simulink model "DriveSystemControl"  (R2023b)
settings: Solver=FixedStepAuto  StartTime=0.0  StopTime=Inf  FixedStep=0.001  RelTol=1e-3
PostLoadFcn:
  | if any(exist('dsrtsu_mdlpostloadfcn', 'file') ~= 0), dsrtsu_mdlpostloadfcn('Execute', bdroot); end
InitFcn:
  | , if any(exist('rtifpga_mdlclblib', 'file') ~= 0), rtifpga_mdlclblib('Init', bdroot); end,
  | , if any(exist('dsmpb_private', 'file') ~= 0), dsmpb_private('dsmpb_mdlclblib', 'Init', bdroot); end,
libraries: dsmpblib x2
(part 4 of 11)

== system DriveSystemControl/Bus Configuration (1) - In/Simulated ECUs/Virya Controller CAN File 08082024/TCU/TX/PDUs/TCU03/sigBPosUndervoltageCutback ==
  ISignal Value : Subsystem
  _sigBPosUndervoltageCutback_ : BusCreator  Inputs=1
  sigBPosUndervoltageCutback : Outport
  wires:
  _sigBPosUndervoltageCutback_/1 -> sigBPosUndervoltageCutback/1  "sigBPosUndervoltageCutback"
  ISignal Value/1(ISignal Value) -> _sigBPosUndervoltageCutback_/1  "ISignal Value"

== system DriveSystemControl/Bus Configuration (1) - In/Simulated ECUs/Virya Controller CAN File 08082024/TCU/TX/PDUs/TCU03/sigBadCalibration ==
  ISignal Value : Subsystem
  _sigBadCalibration_ : BusCreator  Inputs=1
  sigBadCalibration : Outport
  wires:
  _sigBadCalibration_/1 -> sigBadCalibration/1  "sigBadCalibration"
  ISignal Value/1(ISignal Value) -> _sigBadCalibration_/1  "ISignal Value"

== system DriveSystemControl/Bus Configuration (1) - In/Simulated ECUs/Virya Controller CAN File 08082024/TCU/TX/PDUs/TCU03/sigBrakeWiperHigh ==
  ISignal Value : Subsystem
  _sigBrakeWiperHigh_ : BusCreator  Inputs=1
  sigBrakeWiperHigh : Outport
  wires:
  _sigBrakeWiperHigh_/1 -> sigBrakeWiperHigh/1  "sigBrakeWiperHigh"
  ISignal Value/1(ISignal Value) -> _sigBrakeWiperHigh_/1  "ISignal Value"

== system DriveSystemControl/Bus Configuration (1) - In/Simulated ECUs/Virya Controller CAN File 08082024/TCU/TX/PDUs/TCU03/sigBrakeWiperLow ==
  ISignal Value : Subsystem
  _sigBrakeWiperLow_ : BusCreator  Inputs=1
  sigBrakeWiperLow : Outport
  wires:
  _sigBrakeWiperLow_/1 -> sigBrakeWiperLow/1  "sigBrakeWiperLow"
  ISignal Value/1(ISignal Value) -> _sigBrakeWiperLow_/1  "ISignal Value"

== system DriveSystemControl/Bus Configuration (1) - In/Simulated ECUs/Virya Controller CAN File 08082024/TCU/TX/PDUs/TCU03/sigCoil2DriverOpenShort ==
  ISignal Value : Subsystem
  _sigCoil2DriverOpenShort_ : BusCreator  Inputs=1
  sigCoil2DriverOpenShort : Outport
  wires:
  _sigCoil2DriverOpenShort_/1 -> sigCoil2DriverOpenShort/1  "sigCoil2DriverOpenShort"
  ISignal Value/1(ISignal Value) -> _sigCoil2DriverOpenShort_/1  "ISignal Value"

== system DriveSystemControl/Bus Configuration (1) - In/Simulated ECUs/Virya Controller CAN File 08082024/TCU/TX/PDUs/TCU03/sigCoil3DriverOpenShort ==
  ISignal Value : Subsystem
  _sigCoil3DriverOpenShort_ : BusCreator  Inputs=1
  sigCoil3DriverOpenShort : Outport
  wires:
  _sigCoil3DriverOpenShort_/1 -> sigCoil3DriverOpenShort/1  "sigCoil3DriverOpenShort"
  ISignal Value/1(ISignal Value) -> _sigCoil3DriverOpenShort_/1  "ISignal Value"

== system DriveSystemControl/Bus Configuration (1) - In/Simulated ECUs/Virya Controller CAN File 08082024/TCU/TX/PDUs/TCU03/sigCoil4DriverOpenShort ==
  ISignal Value : Subsystem
  _sigCoil4DriverOpenShort_ : BusCreator  Inputs=1
  sigCoil4DriverOpenShort : Outport
  wires:
  _sigCoil4DriverOpenShort_/1 -> sigCoil4DriverOpenShort/1  "sigCoil4DriverOpenShort"
  ISignal Value/1(ISignal Value) -> _sigCoil4DriverOpenShort_/1  "ISignal Value"

== system DriveSystemControl/Bus Configuration (1) - In/Simulated ECUs/Virya Controller CAN File 08082024/TCU/TX/PDUs/TCU03/sigControllerCommonFault ==
  ISignal Value : Subsystem
  _sigControllerCommonFault_ : BusCreator  Inputs=1
  sigControllerCommonFault : Outport
  wires:
  _sigControllerCommonFault_/1 -> sigControllerCommonFault/1  "sigControllerCommonFault"
  ISignal Value/1(ISignal Value) -> _sigControllerCommonFault_/1  "ISignal Value"

== system DriveSystemControl/Bus Configuration (1) - In/Simulated ECUs/Virya Controller CAN File 08082024/TCU/TX/PDUs/TCU03/sigControllerOverCurrent ==
  ISignal Value : Subsystem
  _sigControllerOverCurrent_ : BusCreator  Inputs=1
  sigControllerOverCurrent : Outport
  wires:
  _sigControllerOverCurrent_/1 -> sigControllerOverCurrent/1  "sigControllerOverCurrent"
  ISignal Value/1(ISignal Value) -> _sigControllerOverCurrent_/1  "ISignal Value"

== system DriveSystemControl/Bus Configuration (1) - In/Simulated ECUs/Virya Controller CAN File 08082024/TCU/TX/PDUs/TCU03/sigControllerOvertempCutback ==
  ISignal Value : Subsystem
  _sigControllerOvertempCutback_ : BusCreator  Inputs=1
  sigControllerOvertempCutback : Outport
  wires:
  _sigControllerOvertempCutback_/1 -> sigControllerOvertempCutback/1  "sigControllerOvertempCutback"
  ISignal Value/1(ISignal Value) -> _sigControllerOvertempCutback_/1  "ISignal Value"

== system DriveSystemControl/Bus Configuration (1) - In/Simulated ECUs/Virya Controller CAN File 08082024/TCU/TX/PDUs/TCU03/sigControllerSevereOvertemp ==
  ISignal Value : Subsystem
  _sigControllerSevereOvertemp_ : BusCreator  Inputs=1
  sigControllerSevereOvertemp : Outport
  wires:
  _sigControllerSevereOvertemp_/1 -> sigControllerSevereOvertemp/1  "sigControllerSevereOvertemp"
  ISignal Value/1(ISignal Value) -> _sigControllerSevereOvertemp_/1  "ISignal Value"

== system DriveSystemControl/Bus Configuration (1) - In/Simulated ECUs/Virya Controller CAN File 08082024/TCU/TX/PDUs/TCU03/sigControllerSevereUndertemp ==
  ISignal Value : Subsystem
  _sigControllerSevereUndertemp_ : BusCreator  Inputs=1
  sigControllerSevereUndertemp : Outport
  wires:
  _sigControllerSevereUndertemp_/1 -> sigControllerSevereUndertemp/1  "sigControllerSevereUndertemp"
  ISignal Value/1(ISignal Value) -> _sigControllerSevereUndertemp_/1  "ISignal Value"

== system DriveSystemControl/Bus Configuration (1) - In/Simulated ECUs/Virya Controller CAN File 08082024/TCU/TX/PDUs/TCU03/sigCurrentSensorFault ==
  ISignal Value : Subsystem
  _sigCurrentSensorFault_ : BusCreator  Inputs=1
  sigCurrentSensorFault : Outport
  wires:
  _sigCurrentSensorFault_/1 -> sigCurrentSensorFault/1  "sigCurrentSensorFault"
  ISignal Value/1(ISignal Value) -> _sigCurrentSensorFault_/1  "ISignal Value"

== system DriveSystemControl/Bus Configuration (1) - In/Simulated ECUs/Virya Controller CAN File 08082024/TCU/TX/PDUs/TCU03/sigEEPROMFailure ==
  ISignal Value : Subsystem
  _sigEEPROMFailure_ : BusCreator  Inputs=1
  sigEEPROMFailure : Outport
  wires:
  _sigEEPROMFailure_/1 -> sigEEPROMFailure/1  "sigEEPROMFailure"
  ISignal Value/1(ISignal Value) -> _sigEEPROMFailure_/1  "ISignal Value"

== system DriveSystemControl/Bus Configuration (1) - In/Simulated ECUs/Virya Controller CAN File 08082024/TCU/TX/PDUs/TCU03/sigHighPedalDisable ==
  ISignal Value : Subsystem
  _sigHighPedalDisable_ : BusCreator  Inputs=1
  sigHighPedalDisable : Outport
  wires:
  _sigHighPedalDisable_/1 -> sigHighPedalDisable/1  "sigHighPedalDisable"
  ISignal Value/1(ISignal Value) -> _sigHighPedalDisable_/1  "ISignal Value"

== system DriveSystemControl/Bus Configuration (1) - In/Simulated ECUs/Virya Controller CAN File 08082024/TCU/TX/PDUs/TCU03/sigInsulationResistanceLow ==
  ISignal Value : Subsystem
  _sigInsulationResistanceLow_ : BusCreator  Inputs=1
  sigInsulationResistanceLow : Outport
  wires:
  _sigInsulationResistanceLow_/1 -> sigInsulationResistanceLow/1  "sigInsulationResistanceLow"
  ISignal Value/1(ISignal Value) -> _sigInsulationResistanceLow_/1  "ISignal Value"

== system DriveSystemControl/Bus Configuration (1) - In/Simulated ECUs/Virya Controller CAN File 08082024/TCU/TX/PDUs/TCU03/sigMainContactorWelded ==
  ISignal Value : Subsystem
  _sigMainContactorWelded_ : BusCreator  Inputs=1
  sigMainContactorWelded : Outport
  wires:
  _sigMainContactorWelded_/1 -> sigMainContactorWelded/1  "sigMainContactorWelded"
  ISignal Value/1(ISignal Value) -> _sigMainContactorWelded_/1  "ISignal Value"

== system DriveSystemControl/Bus Configuration (1) - In/Simulated ECUs/Virya Controller CAN File 08082024/TCU/TX/PDUs/TCU03/sigMainContactordidnotClose ==
  ISignal Value : Subsystem
  _sigMainContactordidnotClose_ : BusCreator  Inputs=1
  sigMainContactordidnotClose : Outport
  wires:
  _sigMainContactordidnotClose_/1 -> sigMainContactordidnotClose/1  "sigMainContactordidnotClose"
  ISignal Value/1(ISignal Value) -> _sigMainContactordidnotClose_/1  "ISignal Value"

== system DriveSystemControl/Bus Configuration (1) - In/Simulated ECUs/Virya Controller CAN File 08082024/TCU/TX/PDUs/TCU03/sigMainOpenShort ==
  ISignal Value : Subsystem
  _sigMainOpenShort_ : BusCreator  Inputs=1
  sigMainOpenShort : Outport
  wires:
  _sigMainOpenShort_/1 -> sigMainOpenShort/1  "sigMainOpenShort"
  ISignal Value/1(ISignal Value) -> _sigMainOpenShort_/1  "ISignal Value"

== system DriveSystemControl/Bus Configuration (1) - In/Simulated ECUs/Virya Controller CAN File 08082024/TCU/TX/PDUs/TCU03/sigMotorCharacterization ==
  ISignal Value : Subsystem
  _sigMotorCharacterization_ : BusCreator  Inputs=1
  sigMotorCharacterization : Outport
  wires:
  _sigMotorCharacterization_/1 -> sigMotorCharacterization/1  "sigMotorCharacterization"
  ISignal Value/1(ISignal Value) -> _sigMotorCharacterization_/1  "ISignal Value"

== system DriveSystemControl/Bus Configuration (1) - In/Simulated ECUs/Virya Controller CAN File 08082024/TCU/TX/PDUs/TCU03/sigMotorPhaseOpen ==
  ISignal Value : Subsystem
  _sigMotorPhaseOpen_ : BusCreator  Inputs=1
  sigMotorPhaseOpen : Outport
  wires:
  _sigMotorPhaseOpen_/1 -> sigMotorPhaseOpen/1  "sigMotorPhaseOpen"
  ISignal Value/1(ISignal Value) -> _sigMotorPhaseOpen_/1  "ISignal Value"

== system DriveSystemControl/Bus Configuration (1) - In/Simulated ECUs/Virya Controller CAN File 08082024/TCU/TX/PDUs/TCU03/sigMotorTempHotCutback ==
  ISignal Value : Subsystem
  _sigMotorTempHotCutback_ : BusCreator  Inputs=1
  sigMotorTempHotCutback : Outport
  wires:
  _sigMotorTempHotCutback_/1 -> sigMotorTempHotCutback/1  "sigMotorTempHotCutback"
  ISignal Value/1(ISignal Value) -> _sigMotorTempHotCutback_/1  "ISignal Value"

== system DriveSystemControl/Bus Configuration (1) - In/Simulated ECUs/Virya Controller CAN File 08082024/TCU/TX/PDUs/TCU03/sigMotorTempSensorFault ==
  ISignal Value : Subsystem
  _sigMotorTempSensorFault_ : BusCreator  Inputs=1
  sigMotorTempSensorFault : Outport
  wires:
  _sigMotorTempSensorFault_/1 -> sigMotorTempSensorFault/1  "sigMotorTempSensorFault"
  ISignal Value/1(ISignal Value) -> _sigMotorTempSensorFault_/1  "ISignal Value"

== system DriveSystemControl/Bus Configuration (1) - In/Simulated ECUs/Virya Controller CAN File 08082024/TCU/TX/PDUs/TCU03/sigOEM_BatterySTOPSignal ==
  ISignal Value : Subsystem
  _sigOEM_BatterySTOPSignal_ : BusCreator  Inputs=1
  sigOEM_BatterySTOPSignal : Outport
  wires:
  _sigOEM_BatterySTOPSignal_/1 -> sigOEM_BatterySTOPSignal/1  "sigOEM_BatterySTOPSignal"
  ISignal Value/1(ISignal Value) -> _sigOEM_BatterySTOPSignal_/1  "ISignal Value"

== system DriveSystemControl/Bus Configuration (1) - In/Simulated ECUs/Virya Controller CAN File 08082024/TCU/TX/PDUs/TCU03/sigOEM_NoBatteryCAN ==
  ISignal Value : Subsystem
  _sigOEM_NoBatteryCAN_ : BusCreator  Inputs=1
  sigOEM_NoBatteryCAN : Outport
  wires:
  _sigOEM_NoBatteryCAN_/1 -> sigOEM_NoBatteryCAN/1  "sigOEM_NoBatteryCAN"
  ISignal Value/1(ISignal Value) -> _sigOEM_NoBatteryCAN_/1  "ISignal Value"

== system DriveSystemControl/Bus Configuration (1) - In/Simulated ECUs/Virya Controller CAN File 08082024/TCU/TX/PDUs/TCU03/sigOSGeneral ==
  ISignal Value : Subsystem
  _sigOSGeneral_ : BusCreator  Inputs=1
  sigOSGeneral : Outport
  wires:
  _sigOSGeneral_/1 -> sigOSGeneral/1  "sigOSGeneral"
  ISignal Value/1(ISignal Value) -> _sigOSGeneral_/1  "ISignal Value"

== system DriveSystemControl/Bus Configuration (1) - In/Simulated ECUs/Virya Controller CAN File 08082024/TCU/TX/PDUs/TCU03/sigPMACCommissioningNeeded ==
  ISignal Value : Subsystem
  _sigPMACCommissioningNeeded_ : BusCreator  Inputs=1
  sigPMACCommissioningNeeded : Outport
  wires:
  _sigPMACCommissioningNeeded_/1 -> sigPMACCommissioningNeeded/1  "sigPMACCommissioningNeeded"
  ISignal Value/1(ISignal Value) -> _sigPMACCommissioningNeeded_/1  "ISignal Value"

== system DriveSystemControl/Bus Configuration (1) - In/Simulated ECUs/Virya Controller CAN File 08082024/TCU/TX/PDUs/TCU03/sigParameterChangeFault ==
  ISignal Value : Subsystem
  _sigParameterChangeFault_ : BusCreator  Inputs=1
  sigParameterChangeFault : Outport
  wires:
  _sigParameterChangeFault_/1 -> sigParameterChangeFault/1  "sigParameterChangeFault"
  ISignal Value/1(ISignal Value) -> _sigParameterChangeFault_/1  "ISignal Value"

== system DriveSystemControl/Bus Configuration (1) - In/Simulated ECUs/Virya Controller CAN File 08082024/TCU/TX/PDUs/TCU03/sigPhasePWMMismatch ==
  ISignal Value : Subsystem
  _sigPhasePWMMismatch_ : BusCreator  Inputs=1
  sigPhasePWMMismatch : Outport
  wires:
  _sigPhasePWMMismatch_/1 -> sigPhasePWMMismatch/1  "sigPhasePWMMismatch"
  ISignal Value/1(ISignal Value) -> _sigPhasePWMMismatch_/1  "ISignal Value"

== system DriveSystemControl/Bus Configuration (1) - In/Simulated ECUs/Virya Controller CAN File 08082024/TCU/TX/PDUs/TCU03/sigPrechargeFailed ==
  ISignal Value : Subsystem
  _sigPrechargeFailed_ : BusCreator  Inputs=1
  sigPrechargeFailed : Outport
  wires:
  _sigPrechargeFailed_/1 -> sigPrechargeFailed/1  "sigPrechargeFailed"
  ISignal Value/1(ISignal Value) -> _sigPrechargeFailed_/1  "ISignal Value"

== system DriveSystemControl/Bus Configuration (1) - In/Simulated ECUs/Virya Controller CAN File 08082024/TCU/TX/PDUs/TCU03/sigSevereBPosOvervoltage ==
  ISignal Value : Subsystem
  _sigSevereBPosOvervoltage_ : BusCreator  Inputs=1
  sigSevereBPosOvervoltage : Outport
  wires:
  _sigSevereBPosOvervoltage_/1 -> sigSevereBPosOvervoltage/1  "sigSevereBPosOvervoltage"
  ISignal Value/1(ISignal Value) -> _sigSevereBPosOvervoltage_/1  "ISignal Value"

== system DriveSystemControl/Bus Configuration (1) - In/Simulated ECUs/Virya Controller CAN File 08082024/TCU/TX/PDUs/TCU03/sigSevereBPosUndervoltage ==
  ISignal Value : Subsystem
  _sigSevereBPosUndervoltage_ : BusCreator  Inputs=1
  sigSevereBPosUndervoltage : Outport
  wires:
  _sigSevereBPosUndervoltage_/1 -> sigSevereBPosUndervoltage/1  "sigSevereBPosUndervoltage"
  ISignal Value/1(ISignal Value) -> _sigSevereBPosUndervoltage_/1  "ISignal Value"

== system DriveSystemControl/Bus Configuration (1) - In/Simulated ECUs/Virya Controller CAN File 08082024/TCU/TX/PDUs/TCU03/sigSevereKSIOvervoltage ==
  ISignal Value : Subsystem
  _sigSevereKSIOvervoltage_ : BusCreator  Inputs=1
  sigSevereKSIOvervoltage : Outport
  wires:
  _sigSevereKSIOvervoltage_/1 -> sigSevereKSIOvervoltage/1  "sigSevereKSIOvervoltage"
  ISignal Value/1(ISignal Value) -> _sigSevereKSIOvervoltage_/1  "ISignal Value"

== system DriveSystemControl/Bus Configuration (1) - In/Simulated ECUs/Virya Controller CAN File 08082024/TCU/TX/PDUs/TCU03/sigSevereKSIUndervoltage ==
  ISignal Value : Subsystem
  _sigSevereKSIUndervoltage_ : BusCreator  Inputs=1
  sigSevereKSIUndervoltage : Outport
  wires:
  _sigSevereKSIUndervoltage_/1 -> sigSevereKSIUndervoltage/1  "sigSevereKSIUndervoltage"
  ISignal Value/1(ISignal Value) -> _sigSevereKSIUndervoltage_/1  "ISignal Value"

== system DriveSystemControl/Bus Configuration (1) - In/Simulated ECUs/Virya Controller CAN File 08082024/TCU/TX/PDUs/TCU03/sigSinCosMisalignment ==
  ISignal Value : Subsystem
  _sigSinCosMisalignment_ : BusCreator  Inputs=1
  sigSinCosMisalignment : Outport
  wires:
  _sigSinCosMisalignment_/1 -> sigSinCosMisalignment/1  "sigSinCosMisalignment"
  ISignal Value/1(ISignal Value) -> _sigSinCosMisalignment_/1  "ISignal Value"

== system DriveSystemControl/Bus Configuration (1) - In/Simulated ECUs/Virya Controller CAN File 08082024/TCU/TX/PDUs/TCU03/sigSinCosSensorFault ==
  ISignal Value : Subsystem
  _sigSinCosSensorFault_ : BusCreator  Inputs=1
  sigSinCosSensorFault : Outport
  wires:
  _sigSinCosSensorFault_/1 -> sigSinCosSensorFault/1  "sigSinCosSensorFault"
  ISignal Value/1(ISignal Value) -> _sigSinCosSensorFault_/1  "ISignal Value"

== system DriveSystemControl/Bus Configuration (1) - In/Simulated ECUs/Virya Controller CAN File 08082024/TCU/TX/PDUs/TCU03/sigStallDetected ==
  ISignal Value : Subsystem
  _sigStallDetected_ : BusCreator  Inputs=1
  sigStallDetected : Outport
  wires:
  _sigStallDetected_/1 -> sigStallDetected/1  "sigStallDetected"
  ISignal Value/1(ISignal Value) -> _sigStallDetected_/1  "ISignal Value"

== system DriveSystemControl/Bus Configuration (1) - In/Simulated ECUs/Virya Controller CAN File 08082024/TCU/TX/PDUs/TCU03/sigSupervisorFault ==
  ISignal Value : Subsystem
  _sigSupervisorFault_ : BusCreator  Inputs=1
  sigSupervisorFault : Outport
  wires:
  _sigSupervisorFault_/1 -> sigSupervisorFault/1  "sigSupervisorFault"
  ISignal Value/1(ISignal Value) -> _sigSupervisorFault_/1  "ISignal Value"

== system DriveSystemControl/Bus Configuration (1) - In/Simulated ECUs/Virya Controller CAN File 08082024/TCU/TX/PDUs/TCU03/sigThrottlewiperHigh ==
  ISignal Value : Subsystem
  _sigThrottlewiperHigh_ : BusCreator  Inputs=1
  sigThrottlewiperHigh : Outport
  wires:
  _sigThrottlewiperHigh_/1 -> sigThrottlewiperHigh/1  "sigThrottlewiperHigh"
  ISignal Value/1(ISignal Value) -> _sigThrottlewiperHigh_/1  "ISignal Value"

== system DriveSystemControl/Bus Configuration (1) - In/Simulated ECUs/Virya Controller CAN File 08082024/TCU/TX/PDUs/TCU03/sigThrottlewiperLow ==
  ISignal Value : Subsystem
  _sigThrottlewiperLow_ : BusCreator  Inputs=1
  sigThrottlewiperLow : Outport
  wires:
  _sigThrottlewiperLow_/1 -> sigThrottlewiperLow/1  "sigThrottlewiperLow"
  ISignal Value/1(ISignal Value) -> _sigThrottlewiperLow_/1  "ISignal Value"

== system DriveSystemControl/Bus Configuration (1) - In/Simulated ECUs/Virya Controller CAN File 08082024/TCU/TX/PDUs/TCU03/sigVCLRunTimeError ==
  ISignal Value : Subsystem
  _sigVCLRunTimeError_ : BusCreator  Inputs=1
  sigVCLRunTimeError : Outport
  wires:
  _sigVCLRunTimeError_/1 -> sigVCLRunTimeError/1  "sigVCLRunTimeError"
  ISignal Value/1(ISignal Value) -> _sigVCLRunTimeError_/1  "ISignal Value"

== system DriveSystemControl/Bus Configuration (1) - In/Simulated ECUs/Virya Controller CAN File 08082024/TCU/TX/PDUs/TCU04/sigMCU5_DriveMode ==
  ISignal Value : Subsystem
  _sigMCU5_DriveMode_ : BusCreator  Inputs=1
  sigMCU5_DriveMode : Outport
  wires:
  _sigMCU5_DriveMode_/1 -> sigMCU5_DriveMode/1  "sigMCU5_DriveMode"
  ISignal Value/1(ISignal Value) -> _sigMCU5_DriveMode_/1  "ISignal Value"

== system DriveSystemControl/Bus Configuration (1) - In/Simulated ECUs/Virya Controller CAN File 08082024/TCU/TX/PDUs/TCU04/sigMCU5_Efficiency ==
  ISignal Value : Subsystem
  _sigMCU5_Efficiency_ : BusCreator  Inputs=1
  sigMCU5_Efficiency : Outport
  wires:
  _sigMCU5_Efficiency_/1 -> sigMCU5_Efficiency/1  "sigMCU5_Efficiency"
  ISignal Value/1(ISignal Value) -> _sigMCU5_Efficiency_/1  "ISignal Value"

== system DriveSystemControl/Bus Configuration (1) - In/Simulated ECUs/Virya Controller CAN File 08082024/TCU/TX/PDUs/TCU04/sigMCU5_Hillhold ==
  ISignal Value : Subsystem
  _sigMCU5_Hillhold_ : BusCreator  Inputs=1
  sigMCU5_Hillhold : Outport
  wires:
  _sigMCU5_Hillhold_/1 -> sigMCU5_Hillhold/1  "sigMCU5_Hillhold"
  ISignal Value/1(ISignal Value) -> _sigMCU5_Hillhold_/1  "ISignal Value"

== system DriveSystemControl/Bus Configuration (1) - In/Simulated ECUs/Virya Controller CAN File 08082024/TCU/TX/PDUs/TCU04/sigMCU5_RegenFlag ==
  ISignal Value : Subsystem
  _sigMCU5_RegenFlag_ : BusCreator  Inputs=1
  sigMCU5_RegenFlag : Outport
  wires:
  _sigMCU5_RegenFlag_/1 -> sigMCU5_RegenFlag/1  "sigMCU5_RegenFlag"
  ISignal Value/1(ISignal Value) -> _sigMCU5_RegenFlag_/1  "ISignal Value"

== system DriveSystemControl/Bus Configuration (1) - In/Simulated ECUs/Virya Controller CAN File 08082024/TCU/TX/PDUs/TCU04/sigMCU5_Speed ==
  ISignal Value : Subsystem
  _sigMCU5_Speed_ : BusCreator  Inputs=1
  sigMCU5_Speed : Outport
  wires:
  _sigMCU5_Speed_/1 -> sigMCU5_Speed/1  "sigMCU5_Speed"
  ISignal Value/1(ISignal Value) -> _sigMCU5_Speed_/1  "ISignal Value"

== system DriveSystemControl/Bus Configuration (1) - In/Simulated ECUs/Virya Controller CAN File 08082024/TCU/TX/PDUs/TCU05/sigMCU6_Odometer ==
  ISignal Value : Subsystem
  _sigMCU6_Odometer_ : BusCreator  Inputs=1
  sigMCU6_Odometer : Outport
  wires:
  _sigMCU6_Odometer_/1 -> sigMCU6_Odometer/1  "sigMCU6_Odometer"
  ISignal Value/1(ISignal Value) -> _sigMCU6_Odometer_/1  "ISignal Value"

== system DriveSystemControl/Bus Configuration (1) - Out/Manipulation/Virya Controller CAN File 08082024/WIP/CANChannel/PDUs/BMS01/sigBatteryMalfunctionLight ==
  sigBatteryMalfunctionLight : Inport
  Feature Switch : Subsystem
  _sigBatteryMalfunctionLight_ : BusSelector  OutputSignals=Feature Switch
  wires:
  sigBatteryMalfunctionLight/1 -> _sigBatteryMalfunctionLight_/1  "sigBatteryMalfunctionLight"
  _sigBatteryMalfunctionLight_/1 -> Feature Switch/1(Feature Switch)  "<Feature Switch>"

== system DriveSystemControl/Bus Configuration (1) - Out/Manipulation/Virya Controller CAN File 08082024/WIP/CANChannel/PDUs/BMS01/sigKeyOnIndicator ==
  sigKeyOnIndicator : Inport
  Feature Switch : Subsystem
  _sigKeyOnIndicator_ : BusSelector  OutputSignals=Feature Switch
  wires:
  sigKeyOnIndicator/1 -> _sigKeyOnIndicator_/1  "sigKeyOnIndicator"
  _sigKeyOnIndicator_/1 -> Feature Switch/1(Feature Switch)  "<Feature Switch>"

== system DriveSystemControl/Bus Configuration (1) - Out/Manipulation/Virya Controller CAN File 08082024/WIP/CANChannel/PDUs/BMS01/sigStateOfCharge ==
  sigStateOfCharge : Inport
  Feature Switch : Subsystem
  _sigStateOfCharge_ : BusSelector  OutputSignals=Feature Switch
  wires:
  sigStateOfCharge/1 -> _sigStateOfCharge_/1  "sigStateOfCharge"
  _sigStateOfCharge_/1 -> Feature Switch/1(Feature Switch)  "<Feature Switch>"

== system DriveSystemControl/Bus Configuration (1) - Out/Manipulation/Virya Controller CAN File 08082024/WIP/CANChannel/PDUs/BMS02/sigBatteryCurrent ==
  sigBatteryCurrent : Inport
  Feature Switch : Subsystem
  _sigBatteryCurrent_ : BusSelector  OutputSignals=Feature Switch
  wires:
  sigBatteryCurrent/1 -> _sigBatteryCurrent_/1  "sigBatteryCurrent"
  _sigBatteryCurrent_/1 -> Feature Switch/1(Feature Switch)  "<Feature Switch>"

== system DriveSystemControl/Bus Configuration (1) - Out/Manipulation/Virya Controller CAN File 08082024/WIP/CANChannel/PDUs/BMS02/sigDriveCurrentLimit ==
  sigDriveCurrentLimit : Inport
  Feature Switch : Subsystem
  _sigDriveCurrentLimit_ : BusSelector  OutputSignals=Feature Switch
  wires:
  sigDriveCurrentLimit/1 -> _sigDriveCurrentLimit_/1  "sigDriveCurrentLimit"
  _sigDriveCurrentLimit_/1 -> Feature Switch/1(Feature Switch)  "<Feature Switch>"

== system DriveSystemControl/Bus Configuration (1) - Out/Manipulation/Virya Controller CAN File 08082024/WIP/CANChannel/PDUs/BMS02/sigRegenCurrentLimit ==
  sigRegenCurrentLimit : Inport
  Feature Switch : Subsystem
  _sigRegenCurrentLimit_ : BusSelector  OutputSignals=Feature Switch
  wires:
  sigRegenCurrentLimit/1 -> _sigRegenCurrentLimit_/1  "sigRegenCurrentLimit"
  _sigRegenCurrentLimit_/1 -> Feature Switch/1(Feature Switch)  "<Feature Switch>"

== system DriveSystemControl/Bus Configuration (1) - Out/Manipulation/Virya Controller CAN File 08082024/WIP/CANChannel/PDUs/BMS02/sigVehicleModeRequest ==
  sigVehicleModeRequest : Inport
  Feature Switch : Subsystem
  _sigVehicleModeRequest_ : BusSelector  OutputSignals=Feature Switch
  wires:
  sigVehicleModeRequest/1 -> _sigVehicleModeRequest_/1  "sigVehicleModeRequest"
  _sigVehicleModeRequest_/1 -> Feature Switch/1(Feature Switch)  "<Feature Switch>"

== system DriveSystemControl/Bus Configuration (1) - Out/Manipulation/Virya Controller CAN File 08082024/WIP/CANChannel/PDUs/MainController/CCU_heartBeat ==
  CCU_heartBeat : Inport
  Feature Switch : Subsystem
  _CCU_heartBeat_ : BusSelector  OutputSignals=Feature Switch
  wires:
  CCU_heartBeat/1 -> _CCU_heartBeat_/1  "CCU_heartBeat"
  _CCU_heartBeat_/1 -> Feature Switch/1(Feature Switch)  "<Feature Switch>"

== system DriveSystemControl/Bus Configuration (1) - Out/Manipulation/Virya Controller CAN File 08082024/WIP/CANChannel/PDUs/MainController/notUsed ==
  notUsed : Inport
  Feature Switch : Subsystem
  _notUsed_ : BusSelector  OutputSignals=Feature Switch
  wires:
  notUsed/1 -> _notUsed_/1  "notUsed"
  _notUsed_/1 -> Feature Switch/1(Feature Switch)  "<Feature Switch>"

== system DriveSystemControl/Bus Configuration (1) - Out/Manipulation/Virya Controller CAN File 08082024/WIP/CANChannel/PDUs/MainController/setAutoParkBreak ==
  setAutoParkBreak : Inport
  Feature Switch : Subsystem
  _setAutoParkBreak_ : BusSelector  OutputSignals=Feature Switch
  wires:
  setAutoParkBreak/1 -> _setAutoParkBreak_/1  "setAutoParkBreak"
  _setAutoParkBreak_/1 -> Feature Switch/1(Feature Switch)  "<Feature Switch>"

== system DriveSystemControl/Bus Configuration (1) - Out/Manipulation/Virya Controller CAN File 08082024/WIP/CANChannel/PDUs/MainController/setBreake ==
  setBreake : Inport
  Feature Switch : Subsystem
  _setBreake_ : BusSelector  OutputSignals=Feature Switch
  wires:
  setBreake/1 -> _setBreake_/1  "setBreake"
  _setBreake_/1 -> Feature Switch/1(Feature Switch)  "<Feature Switch>"

== system DriveSystemControl/Bus Configuration (1) - Out/Manipulation/Virya Controller CAN File 08082024/WIP/CANChannel/PDUs/MainController/setDirection ==
  setDirection : Inport
  Feature Switch : Subsystem
  _setDirection_ : BusSelector  OutputSignals=Feature Switch
  wires:
  setDirection/1 -> _setDirection_/1  "setDirection"
  _setDirection_/1 -> Feature Switch/1(Feature Switch)  "<Feature Switch>"

== system DriveSystemControl/Bus Configuration (1) - Out/Manipulation/Virya Controller CAN File 08082024/WIP/CANChannel/PDUs/MainController/setDriveMode ==
  setDriveMode : Inport
  Feature Switch : Subsystem
  _setDriveMode_ : BusSelector  OutputSignals=Feature Switch
  wires:
  setDriveMode/1 -> _setDriveMode_/1  "setDriveMode"
  _setDriveMode_/1 -> Feature Switch/1(Feature Switch)  "<Feature Switch>"

== system DriveSystemControl/Bus Configuration (1) - Out/Manipulation/Virya Controller CAN File 08082024/WIP/CANChannel/PDUs/MainController/setVelocity ==
  setVelocity : Inport
  Feature Switch : Subsystem
  _setVelocity_ : BusSelector  OutputSignals=Feature Switch
  wires:
  setVelocity/1 -> _setVelocity_/1  "setVelocity"
  _setVelocity_/1 -> Feature Switch/1(Feature Switch)  "<Feature Switch>"

== system DriveSystemControl/Bus Configuration (1) - Out/Manipulation/Virya Controller CAN File 08082024/WIP/CANChannel/PDUs/MainController/steeringPower ==
  steeringPower : Inport
  Feature Switch : Subsystem
  _steeringPower_ : BusSelector  OutputSignals=Feature Switch
  wires:
  steeringPower/1 -> _steeringPower_/1  "steeringPower"
  _steeringPower_/1 -> Feature Switch/1(Feature Switch)  "<Feature Switch>"

== system DriveSystemControl/Bus Configuration (1) - Out/Manipulation/Virya Controller CAN File 08082024/WIP/CANChannel/PDUs/TCU01/sigBrake ==
  sigBrake : Inport
  Feature Switch : Subsystem
  _sigBrake_ : BusSelector  OutputSignals=Feature Switch
  wires:
  sigBrake/1 -> _sigBrake_/1  "sigBrake"
  _sigBrake_/1 -> Feature Switch/1(Feature Switch)  "<Feature Switch>"

== system DriveSystemControl/Bus Configuration (1) - Out/Manipulation/Virya Controller CAN File 08082024/WIP/CANChannel/PDUs/TCU01/sigControllerTemperature ==
  sigControllerTemperature : Inport
  Feature Switch : Subsystem
  _sigControllerTemperature_ : BusSelector  OutputSignals=Feature Switch
  wires:
  sigControllerTemperature/1 -> _sigControllerTemperature_/1  "sigControllerTemperature"
  _sigControllerTemperature_/1 -> Feature Switch/1(Feature Switch)  "<Feature Switch>"

== system DriveSystemControl/Bus Configuration (1) - Out/Manipulation/Virya Controller CAN File 08082024/WIP/CANChannel/PDUs/TCU01/sigDriveMode ==
  sigDriveMode : Inport
  Feature Switch : Subsystem
  _sigDriveMode_ : BusSelector  OutputSignals=Feature Switch
  wires:
  sigDriveMode/1 -> _sigDriveMode_/1  "sigDriveMode"
  _sigDriveMode_/1 -> Feature Switch/1(Feature Switch)  "<Feature Switch>"

== system DriveSystemControl/Bus Configuration (1) - Out/Manipulation/Virya Controller CAN File 08082024/WIP/CANChannel/PDUs/TCU01/sigMotorTemperature ==
  sigMotorTemperature : Inport
  Feature Switch : Subsystem
  _sigMotorTemperature_ : BusSelector  OutputSignals=Feature Switch
  wires:
  sigMotorTemperature/1 -> _sigMotorTemperature_/1  "sigMotorTemperature"
  _sigMotorTemperature_/1 -> Feature Switch/1(Feature Switch)  "<Feature Switch>"

== system DriveSystemControl/Bus Configuration (1) - Out/Manipulation/Virya Controller CAN File 08082024/WIP/CANChannel/PDUs/TCU01/sigRMSCurrent ==
  sigRMSCurrent : Inport
  Feature Switch : Subsystem
  _sigRMSCurrent_ : BusSelector  OutputSignals=Feature Switch
  wires:
  sigRMSCurrent/1 -> _sigRMSCurrent_/1  "sigRMSCurrent"
  _sigRMSCurrent_/1 -> Feature Switch/1(Feature Switch)  "<Feature Switch>"

== system DriveSystemControl/Bus Configuration (1) - Out/Manipulation/Virya Controller CAN File 08082024/WIP/CANChannel/PDUs/TCU01/sigSpeed ==
  sigSpeed : Inport
  Feature Switch : Subsystem
  _sigSpeed_ : BusSelector  OutputSignals=Feature Switch
  wires:
  sigSpeed/1 -> _sigSpeed_/1  "sigSpeed"
  _sigSpeed_/1 -> Feature Switch/1(Feature Switch)  "<Feature Switch>"

== system DriveSystemControl/Bus Configuration (1) - Out/Manipulation/Virya Controller CAN File 08082024/WIP/CANChannel/PDUs/TCU01/sigThrottle ==
  sigThrottle : Inport
  Feature Switch : Subsystem
  _sigThrottle_ : BusSelector  OutputSignals=Feature Switch
  wires:
  sigThrottle/1 -> _sigThrottle_/1  "sigThrottle"
  _sigThrottle_/1 -> Feature Switch/1(Feature Switch)  "<Feature Switch>"

== system DriveSystemControl/Bus Configuration (1) - Out/Manipulation/Virya Controller CAN File 08082024/WIP/CANChannel/PDUs/TCU02/sigCapacitorVoltage ==
  sigCapacitorVoltage : Inport
  Feature Switch : Subsystem
  _sigCapacitorVoltage_ : BusSelector  OutputSignals=Feature Switch
  wires:
  sigCapacitorVoltage/1 -> _sigCapacitorVoltage_/1  "sigCapacitorVoltage"
  _sigCapacitorVoltage_/1 -> Feature Switch/1(Feature Switch)  "<Feature Switch>"

== system DriveSystemControl/Bus Configuration (1) - Out/Manipulation/Virya Controller CAN File 08082024/WIP/CANChannel/PDUs/TCU02/sigMotorRPM ==
  sigMotorRPM : Inport
  Feature Switch : Subsystem
  _sigMotorRPM_ : BusSelector  OutputSignals=Feature Switch
  wires:
  sigMotorRPM/1 -> _sigMotorRPM_/1  "sigMotorRPM"
  _sigMotorRPM_/1 -> Feature Switch/1(Feature Switch)  "<Feature Switch>"

== system DriveSystemControl/Bus Configuration (1) - Out/Manipulation/Virya Controller CAN File 08082024/WIP/CANChannel/PDUs/TCU02/sigOdometer ==
  sigOdometer : Inport
  Feature Switch : Subsystem
  _sigOdometer_ : BusSelector  OutputSignals=Feature Switch
  wires:
  sigOdometer/1 -> _sigOdometer_/1  "sigOdometer"
  _sigOdometer_/1 -> Feature Switch/1(Feature Switch)  "<Feature Switch>"

== system DriveSystemControl/Bus Configuration (1) - Out/Manipulation/Virya Controller CAN File 08082024/WIP/CANChannel/PDUs/TCU03/Controller_CompleteFaults ==
  Controller_CompleteFaults : Inport
  Feature Switch : Subsystem
  _Controller_CompleteFaults_ : BusSelector  OutputSignals=Feature Switch
  wires:
  Controller_CompleteFaults/1 -> _Controller_CompleteFaults_/1  "Controller_CompleteFaults"
  _Controller_CompleteFaults_/1 -> Feature Switch/1(Feature Switch)  "<Feature Switch>"

== system DriveSystemControl/Bus Configuration (1) - Out/Manipulation/Virya Controller CAN File 08082024/WIP/CANChannel/PDUs/TCU03/sig5VSupplyFailure ==
  sig5VSupplyFailure : Inport
  Feature Switch : Subsystem
  _sig5VSupplyFailure_ : BusSelector  OutputSignals=Feature Switch
  wires:
  sig5VSupplyFailure/1 -> _sig5VSupplyFailure_/1  "sig5VSupplyFailure"
  _sig5VSupplyFailure_/1 -> Feature Switch/1(Feature Switch)  "<Feature Switch>"

== system DriveSystemControl/Bus Configuration (1) - Out/Manipulation/Virya Controller CAN File 08082024/WIP/CANChannel/PDUs/TCU03/sigBPosOvervoltageCutback ==
  sigBPosOvervoltageCutback : Inport
  Feature Switch : Subsystem
  _sigBPosOvervoltageCutback_ : BusSelector  OutputSignals=Feature Switch
  wires:
  sigBPosOvervoltageCutback/1 -> _sigBPosOvervoltageCutback_/1  "sigBPosOvervoltageCutback"
  _sigBPosOvervoltageCutback_/1 -> Feature Switch/1(Feature Switch)  "<Feature Switch>"

== system DriveSystemControl/Bus Configuration (1) - Out/Manipulation/Virya Controller CAN File 08082024/WIP/CANChannel/PDUs/TCU03/sigBPosUndervoltageCutback ==
  sigBPosUndervoltageCutback : Inport
  Feature Switch : Subsystem
  _sigBPosUndervoltageCutback_ : BusSelector  OutputSignals=Feature Switch
  wires:
  sigBPosUndervoltageCutback/1 -> _sigBPosUndervoltageCutback_/1  "sigBPosUndervoltageCutback"
  _sigBPosUndervoltageCutback_/1 -> Feature Switch/1(Feature Switch)  "<Feature Switch>"

== system DriveSystemControl/Bus Configuration (1) - Out/Manipulation/Virya Controller CAN File 08082024/WIP/CANChannel/PDUs/TCU03/sigBadCalibration ==
  sigBadCalibration : Inport
  Feature Switch : Subsystem
  _sigBadCalibration_ : BusSelector  OutputSignals=Feature Switch
  wires:
  sigBadCalibration/1 -> _sigBadCalibration_/1  "sigBadCalibration"
  _sigBadCalibration_/1 -> Feature Switch/1(Feature Switch)  "<Feature Switch>"

== system DriveSystemControl/Bus Configuration (1) - Out/Manipulation/Virya Controller CAN File 08082024/WIP/CANChannel/PDUs/TCU03/sigBrakeWiperHigh ==
  sigBrakeWiperHigh : Inport
  Feature Switch : Subsystem
  _sigBrakeWiperHigh_ : BusSelector  OutputSignals=Feature Switch
  wires:
  sigBrakeWiperHigh/1 -> _sigBrakeWiperHigh_/1  "sigBrakeWiperHigh"
  _sigBrakeWiperHigh_/1 -> Feature Switch/1(Feature Switch)  "<Feature Switch>"

== system DriveSystemControl/Bus Configuration (1) - Out/Manipulation/Virya Controller CAN File 08082024/WIP/CANChannel/PDUs/TCU03/sigBrakeWiperLow ==
  sigBrakeWiperLow : Inport
  Feature Switch : Subsystem
  _sigBrakeWiperLow_ : BusSelector  OutputSignals=Feature Switch
  wires:
  sigBrakeWiperLow/1 -> _sigBrakeWiperLow_/1  "sigBrakeWiperLow"
  _sigBrakeWiperLow_/1 -> Feature Switch/1(Feature Switch)  "<Feature Switch>"

== system DriveSystemControl/Bus Configuration (1) - Out/Manipulation/Virya Controller CAN File 08082024/WIP/CANChannel/PDUs/TCU03/sigCoil2DriverOpenShort ==
  sigCoil2DriverOpenShort : Inport
  Feature Switch : Subsystem
  _sigCoil2DriverOpenShort_ : BusSelector  OutputSignals=Feature Switch
  wires:
  sigCoil2DriverOpenShort/1 -> _sigCoil2DriverOpenShort_/1  "sigCoil2DriverOpenShort"
  _sigCoil2DriverOpenShort_/1 -> Feature Switch/1(Feature Switch)  "<Feature Switch>"

== system DriveSystemControl/Bus Configuration (1) - Out/Manipulation/Virya Controller CAN File 08082024/WIP/CANChannel/PDUs/TCU03/sigCoil3DriverOpenShort ==
  sigCoil3DriverOpenShort : Inport
  Feature Switch : Subsystem
  _sigCoil3DriverOpenShort_ : BusSelector  OutputSignals=Feature Switch
  wires:
  sigCoil3DriverOpenShort/1 -> _sigCoil3DriverOpenShort_/1  "sigCoil3DriverOpenShort"
  _sigCoil3DriverOpenShort_/1 -> Feature Switch/1(Feature Switch)  "<Feature Switch>"

== system DriveSystemControl/Bus Configuration (1) - Out/Manipulation/Virya Controller CAN File 08082024/WIP/CANChannel/PDUs/TCU03/sigCoil4DriverOpenShort ==
  sigCoil4DriverOpenShort : Inport
  Feature Switch : Subsystem
  _sigCoil4DriverOpenShort_ : BusSelector  OutputSignals=Feature Switch
  wires:
  sigCoil4DriverOpenShort/1 -> _sigCoil4DriverOpenShort_/1  "sigCoil4DriverOpenShort"
  _sigCoil4DriverOpenShort_/1 -> Feature Switch/1(Feature Switch)  "<Feature Switch>"

== system DriveSystemControl/Bus Configuration (1) - Out/Manipulation/Virya Controller CAN File 08082024/WIP/CANChannel/PDUs/TCU03/sigControllerCommonFault ==
  sigControllerCommonFault : Inport
  Feature Switch : Subsystem
  _sigControllerCommonFault_ : BusSelector  OutputSignals=Feature Switch
  wires:
  sigControllerCommonFault/1 -> _sigControllerCommonFault_/1  "sigControllerCommonFault"
  _sigControllerCommonFault_/1 -> Feature Switch/1(Feature Switch)  "<Feature Switch>"

== system DriveSystemControl/Bus Configuration (1) - Out/Manipulation/Virya Controller CAN File 08082024/WIP/CANChannel/PDUs/TCU03/sigControllerOverCurrent ==
  sigControllerOverCurrent : Inport
  Feature Switch : Subsystem
  _sigControllerOverCurrent_ : BusSelector  OutputSignals=Feature Switch
  wires:
  sigControllerOverCurrent/1 -> _sigControllerOverCurrent_/1  "sigControllerOverCurrent"
  _sigControllerOverCurrent_/1 -> Feature Switch/1(Feature Switch)  "<Feature Switch>"

== system DriveSystemControl/Bus Configuration (1) - Out/Manipulation/Virya Controller CAN File 08082024/WIP/CANChannel/PDUs/TCU03/sigControllerOvertempCutback ==
  sigControllerOvertempCutback : Inport
  Feature Switch : Subsystem
  _sigControllerOvertempCutback_ : BusSelector  OutputSignals=Feature Switch
  wires:
  sigControllerOvertempCutback/1 -> _sigControllerOvertempCutback_/1  "sigControllerOvertempCutback"
  _sigControllerOvertempCutback_/1 -> Feature Switch/1(Feature Switch)  "<Feature Switch>"

== system DriveSystemControl/Bus Configuration (1) - Out/Manipulation/Virya Controller CAN File 08082024/WIP/CANChannel/PDUs/TCU03/sigControllerSevereOvertemp ==
  sigControllerSevereOvertemp : Inport
  Feature Switch : Subsystem
  _sigControllerSevereOvertemp_ : BusSelector  OutputSignals=Feature Switch
  wires:
  sigControllerSevereOvertemp/1 -> _sigControllerSevereOvertemp_/1  "sigControllerSevereOvertemp"
  _sigControllerSevereOvertemp_/1 -> Feature Switch/1(Feature Switch)  "<Feature Switch>"

== system DriveSystemControl/Bus Configuration (1) - Out/Manipulation/Virya Controller CAN File 08082024/WIP/CANChannel/PDUs/TCU03/sigControllerSevereUndertemp ==
  sigControllerSevereUndertemp : Inport
  Feature Switch : Subsystem
  _sigControllerSevereUndertemp_ : BusSelector  OutputSignals=Feature Switch
  wires:
  sigControllerSevereUndertemp/1 -> _sigControllerSevereUndertemp_/1  "sigControllerSevereUndertemp"
  _sigControllerSevereUndertemp_/1 -> Feature Switch/1(Feature Switch)  "<Feature Switch>"

== system DriveSystemControl/Bus Configuration (1) - Out/Manipulation/Virya Controller CAN File 08082024/WIP/CANChannel/PDUs/TCU03/sigCurrentSensorFault ==
  sigCurrentSensorFault : Inport
  Feature Switch : Subsystem
  _sigCurrentSensorFault_ : BusSelector  OutputSignals=Feature Switch
  wires:
  sigCurrentSensorFault/1 -> _sigCurrentSensorFault_/1  "sigCurrentSensorFault"
  _sigCurrentSensorFault_/1 -> Feature Switch/1(Feature Switch)  "<Feature Switch>"

== system DriveSystemControl/Bus Configuration (1) - Out/Manipulation/Virya Controller CAN File 08082024/WIP/CANChannel/PDUs/TCU03/sigEEPROMFailure ==
  sigEEPROMFailure : Inport
  Feature Switch : Subsystem
  _sigEEPROMFailure_ : BusSelector  OutputSignals=Feature Switch
  wires:
  sigEEPROMFailure/1 -> _sigEEPROMFailure_/1  "sigEEPROMFailure"
  _sigEEPROMFailure_/1 -> Feature Switch/1(Feature Switch)  "<Feature Switch>"

== system DriveSystemControl/Bus Configuration (1) - Out/Manipulation/Virya Controller CAN File 08082024/WIP/CANChannel/PDUs/TCU03/sigHighPedalDisable ==
  sigHighPedalDisable : Inport
  Feature Switch : Subsystem
  _sigHighPedalDisable_ : BusSelector  OutputSignals=Feature Switch
  wires:
  sigHighPedalDisable/1 -> _sigHighPedalDisable_/1  "sigHighPedalDisable"
  _sigHighPedalDisable_/1 -> Feature Switch/1(Feature Switch)  "<Feature Switch>"

== system DriveSystemControl/Bus Configuration (1) - Out/Manipulation/Virya Controller CAN File 08082024/WIP/CANChannel/PDUs/TCU03/sigInsulationResistanceLow ==
  sigInsulationResistanceLow : Inport
  Feature Switch : Subsystem
  _sigInsulationResistanceLow_ : BusSelector  OutputSignals=Feature Switch
  wires:
  sigInsulationResistanceLow/1 -> _sigInsulationResistanceLow_/1  "sigInsulationResistanceLow"
  _sigInsulationResistanceLow_/1 -> Feature Switch/1(Feature Switch)  "<Feature Switch>"

== system DriveSystemControl/Bus Configuration (1) - Out/Manipulation/Virya Controller CAN File 08082024/WIP/CANChannel/PDUs/TCU03/sigMainContactorWelded ==
  sigMainContactorWelded : Inport
  Feature Switch : Subsystem
  _sigMainContactorWelded_ : BusSelector  OutputSignals=Feature Switch
  wires:
  sigMainContactorWelded/1 -> _sigMainContactorWelded_/1  "sigMainContactorWelded"
  _sigMainContactorWelded_/1 -> Feature Switch/1(Feature Switch)  "<Feature Switch>"

== system DriveSystemControl/Bus Configuration (1) - Out/Manipulation/Virya Controller CAN File 08082024/WIP/CANChannel/PDUs/TCU03/sigMainContactordidnotClose ==
  sigMainContactordidnotClose : Inport
  Feature Switch : Subsystem
  _sigMainContactordidnotClose_ : BusSelector  OutputSignals=Feature Switch
  wires:
  sigMainContactordidnotClose/1 -> _sigMainContactordidnotClose_/1  "sigMainContactordidnotClose"
  _sigMainContactordidnotClose_/1 -> Feature Switch/1(Feature Switch)  "<Feature Switch>"

== system DriveSystemControl/Bus Configuration (1) - Out/Manipulation/Virya Controller CAN File 08082024/WIP/CANChannel/PDUs/TCU03/sigMainOpenShort ==
  sigMainOpenShort : Inport
  Feature Switch : Subsystem
  _sigMainOpenShort_ : BusSelector  OutputSignals=Feature Switch
  wires:
  sigMainOpenShort/1 -> _sigMainOpenShort_/1  "sigMainOpenShort"
  _sigMainOpenShort_/1 -> Feature Switch/1(Feature Switch)  "<Feature Switch>"

== system DriveSystemControl/Bus Configuration (1) - Out/Manipulation/Virya Controller CAN File 08082024/WIP/CANChannel/PDUs/TCU03/sigMotorCharacterization ==
  sigMotorCharacterization : Inport
  Feature Switch : Subsystem
  _sigMotorCharacterization_ : BusSelector  OutputSignals=Feature Switch
  wires:
  sigMotorCharacterization/1 -> _sigMotorCharacterization_/1  "sigMotorCharacterization"
  _sigMotorCharacterization_/1 -> Feature Switch/1(Feature Switch)  "<Feature Switch>"

== system DriveSystemControl/Bus Configuration (1) - Out/Manipulation/Virya Controller CAN File 08082024/WIP/CANChannel/PDUs/TCU03/sigMotorPhaseOpen ==
  sigMotorPhaseOpen : Inport
  Feature Switch : Subsystem
  _sigMotorPhaseOpen_ : BusSelector  OutputSignals=Feature Switch
  wires:
  sigMotorPhaseOpen/1 -> _sigMotorPhaseOpen_/1  "sigMotorPhaseOpen"
  _sigMotorPhaseOpen_/1 -> Feature Switch/1(Feature Switch)  "<Feature Switch>"

== system DriveSystemControl/Bus Configuration (1) - Out/Manipulation/Virya Controller CAN File 08082024/WIP/CANChannel/PDUs/TCU03/sigMotorTempHotCutback ==
  sigMotorTempHotCutback : Inport
  Feature Switch : Subsystem
  _sigMotorTempHotCutback_ : BusSelector  OutputSignals=Feature Switch
  wires:
  sigMotorTempHotCutback/1 -> _sigMotorTempHotCutback_/1  "sigMotorTempHotCutback"
  _sigMotorTempHotCutback_/1 -> Feature Switch/1(Feature Switch)  "<Feature Switch>"

== system DriveSystemControl/Bus Configuration (1) - Out/Manipulation/Virya Controller CAN File 08082024/WIP/CANChannel/PDUs/TCU03/sigMotorTempSensorFault ==
  sigMotorTempSensorFault : Inport
  Feature Switch : Subsystem
  _sigMotorTempSensorFault_ : BusSelector  OutputSignals=Feature Switch
  wires:
  sigMotorTempSensorFault/1 -> _sigMotorTempSensorFault_/1  "sigMotorTempSensorFault"
  _sigMotorTempSensorFault_/1 -> Feature Switch/1(Feature Switch)  "<Feature Switch>"

== system DriveSystemControl/Bus Configuration (1) - Out/Manipulation/Virya Controller CAN File 08082024/WIP/CANChannel/PDUs/TCU03/sigOEM_BatterySTOPSignal ==
  sigOEM_BatterySTOPSignal : Inport
  Feature Switch : Subsystem
  _sigOEM_BatterySTOPSignal_ : BusSelector  OutputSignals=Feature Switch
  wires:
  sigOEM_BatterySTOPSignal/1 -> _sigOEM_BatterySTOPSignal_/1  "sigOEM_BatterySTOPSignal"
  _sigOEM_BatterySTOPSignal_/1 -> Feature Switch/1(Feature Switch)  "<Feature Switch>"

== system DriveSystemControl/Bus Configuration (1) - Out/Manipulation/Virya Controller CAN File 08082024/WIP/CANChannel/PDUs/TCU03/sigOEM_NoBatteryCAN ==
  sigOEM_NoBatteryCAN : Inport
  Feature Switch : Subsystem
  _sigOEM_NoBatteryCAN_ : BusSelector  OutputSignals=Feature Switch
  wires:
  sigOEM_NoBatteryCAN/1 -> _sigOEM_NoBatteryCAN_/1  "sigOEM_NoBatteryCAN"
  _sigOEM_NoBatteryCAN_/1 -> Feature Switch/1(Feature Switch)  "<Feature Switch>"

== system DriveSystemControl/Bus Configuration (1) - Out/Manipulation/Virya Controller CAN File 08082024/WIP/CANChannel/PDUs/TCU03/sigOSGeneral ==
  sigOSGeneral : Inport
  Feature Switch : Subsystem
  _sigOSGeneral_ : BusSelector  OutputSignals=Feature Switch
  wires:
  sigOSGeneral/1 -> _sigOSGeneral_/1  "sigOSGeneral"
  _sigOSGeneral_/1 -> Feature Switch/1(Feature Switch)  "<Feature Switch>"

== system DriveSystemControl/Bus Configuration (1) - Out/Manipulation/Virya Controller CAN File 08082024/WIP/CANChannel/PDUs/TCU03/sigPMACCommissioningNeeded ==
  sigPMACCommissioningNeeded : Inport
  Feature Switch : Subsystem
  _sigPMACCommissioningNeeded_ : BusSelector  OutputSignals=Feature Switch
  wires:
  sigPMACCommissioningNeeded/1 -> _sigPMACCommissioningNeeded_/1  "sigPMACCommissioningNeeded"
  _sigPMACCommissioningNeeded_/1 -> Feature Switch/1(Feature Switch)  "<Feature Switch>"

== system DriveSystemControl/Bus Configuration (1) - Out/Manipulation/Virya Controller CAN File 08082024/WIP/CANChannel/PDUs/TCU03/sigParameterChangeFault ==
  sigParameterChangeFault : Inport
  Feature Switch : Subsystem
  _sigParameterChangeFault_ : BusSelector  OutputSignals=Feature Switch
  wires:
  sigParameterChangeFault/1 -> _sigParameterChangeFault_/1  "sigParameterChangeFault"
  _sigParameterChangeFault_/1 -> Feature Switch/1(Feature Switch)  "<Feature Switch>"

== system DriveSystemControl/Bus Configuration (1) - Out/Manipulation/Virya Controller CAN File 08082024/WIP/CANChannel/PDUs/TCU03/sigPhasePWMMismatch ==
  sigPhasePWMMismatch : Inport
  Feature Switch : Subsystem
  _sigPhasePWMMismatch_ : BusSelector  OutputSignals=Feature Switch
  wires:
  sigPhasePWMMismatch/1 -> _sigPhasePWMMismatch_/1  "sigPhasePWMMismatch"
  _sigPhasePWMMismatch_/1 -> Feature Switch/1(Feature Switch)  "<Feature Switch>"

== system DriveSystemControl/Bus Configuration (1) - Out/Manipulation/Virya Controller CAN File 08082024/WIP/CANChannel/PDUs/TCU03/sigPrechargeFailed ==
  sigPrechargeFailed : Inport
  Feature Switch : Subsystem
  _sigPrechargeFailed_ : BusSelector  OutputSignals=Feature Switch
  wires:
  sigPrechargeFailed/1 -> _sigPrechargeFailed_/1  "sigPrechargeFailed"
  _sigPrechargeFailed_/1 -> Feature Switch/1(Feature Switch)  "<Feature Switch>"

== system DriveSystemControl/Bus Configuration (1) - Out/Manipulation/Virya Controller CAN File 08082024/WIP/CANChannel/PDUs/TCU03/sigSevereBPosOvervoltage ==
  sigSevereBPosOvervoltage : Inport
  Feature Switch : Subsystem
  _sigSevereBPosOvervoltage_ : BusSelector  OutputSignals=Feature Switch
  wires:
  sigSevereBPosOvervoltage/1 -> _sigSevereBPosOvervoltage_/1  "sigSevereBPosOvervoltage"
  _sigSevereBPosOvervoltage_/1 -> Feature Switch/1(Feature Switch)  "<Feature Switch>"

== system DriveSystemControl/Bus Configuration (1) - Out/Manipulation/Virya Controller CAN File 08082024/WIP/CANChannel/PDUs/TCU03/sigSevereBPosUndervoltage ==
  sigSevereBPosUndervoltage : Inport
  Feature Switch : Subsystem
  _sigSevereBPosUndervoltage_ : BusSelector  OutputSignals=Feature Switch
  wires:
  sigSevereBPosUndervoltage/1 -> _sigSevereBPosUndervoltage_/1  "sigSevereBPosUndervoltage"
  _sigSevereBPosUndervoltage_/1 -> Feature Switch/1(Feature Switch)  "<Feature Switch>"

== system DriveSystemControl/Bus Configuration (1) - Out/Manipulation/Virya Controller CAN File 08082024/WIP/CANChannel/PDUs/TCU03/sigSevereKSIOvervoltage ==
  sigSevereKSIOvervoltage : Inport
  Feature Switch : Subsystem
  _sigSevereKSIOvervoltage_ : BusSelector  OutputSignals=Feature Switch
  wires:
  sigSevereKSIOvervoltage/1 -> _sigSevereKSIOvervoltage_/1  "sigSevereKSIOvervoltage"
  _sigSevereKSIOvervoltage_/1 -> Feature Switch/1(Feature Switch)  "<Feature Switch>"

== system DriveSystemControl/Bus Configuration (1) - Out/Manipulation/Virya Controller CAN File 08082024/WIP/CANChannel/PDUs/TCU03/sigSevereKSIUndervoltage ==
  sigSevereKSIUndervoltage : Inport
  Feature Switch : Subsystem
  _sigSevereKSIUndervoltage_ : BusSelector  OutputSignals=Feature Switch
  wires:
  sigSevereKSIUndervoltage/1 -> _sigSevereKSIUndervoltage_/1  "sigSevereKSIUndervoltage"
  _sigSevereKSIUndervoltage_/1 -> Feature Switch/1(Feature Switch)  "<Feature Switch>"

== system DriveSystemControl/Bus Configuration (1) - Out/Manipulation/Virya Controller CAN File 08082024/WIP/CANChannel/PDUs/TCU03/sigSinCosMisalignment ==
  sigSinCosMisalignment : Inport
  Feature Switch : Subsystem
  _sigSinCosMisalignment_ : BusSelector  OutputSignals=Feature Switch
  wires:
  sigSinCosMisalignment/1 -> _sigSinCosMisalignment_/1  "sigSinCosMisalignment"
  _sigSinCosMisalignment_/1 -> Feature Switch/1(Feature Switch)  "<Feature Switch>"

== system DriveSystemControl/Bus Configuration (1) - Out/Manipulation/Virya Controller CAN File 08082024/WIP/CANChannel/PDUs/TCU03/sigSinCosSensorFault ==
  sigSinCosSensorFault : Inport
  Feature Switch : Subsystem
  _sigSinCosSensorFault_ : BusSelector  OutputSignals=Feature Switch
  wires:
  sigSinCosSensorFault/1 -> _sigSinCosSensorFault_/1  "sigSinCosSensorFault"
  _sigSinCosSensorFault_/1 -> Feature Switch/1(Feature Switch)  "<Feature Switch>"

== system DriveSystemControl/Bus Configuration (1) - Out/Manipulation/Virya Controller CAN File 08082024/WIP/CANChannel/PDUs/TCU03/sigStallDetected ==
  sigStallDetected : Inport
  Feature Switch : Subsystem
  _sigStallDetected_ : BusSelector  OutputSignals=Feature Switch
  wires:
  sigStallDetected/1 -> _sigStallDetected_/1  "sigStallDetected"
  _sigStallDetected_/1 -> Feature Switch/1(Feature Switch)  "<Feature Switch>"
